simulink model "chart"  (R2020b)
settings: Solver=FixedStepDiscrete  StartTime=0.0  StopTime=10.0  FixedStep=0.1  RelTol=1e-3  EnableMultiTasking=on
settings Model: Creator=Admin  LastModifiedBy=Admin
settings SolverCC: AutoInsertRateTranBlk=on
settings DataIOCC: LimitDataPoints=on
settings OptimizationCC: LifeSpan=inf
settings DebuggingCC: AllowSymbolicDim=off  SFUnexpectedBacktrackingDiag=warning  SFNoUnconditionalDefaultTransitionDiag=warning  SFExecutionAtInitializationDiag=none  ArithmeticOperatorsInVariantConditions=warning
settings SFSimCC: SimUseLocalCustomCode=off  CustomCodeUndefinedFunction=UseInterfaceOnly
settings RTWCC: RTWUseLocalCustomCode=off
settings CodeAppCC: StateflowObjectComments=on
settings GRTTargetCC: TargetLangStandard=C89/C90 (ANSI)
settings ConfigComp: CovMetricSettings=dw  CovSaveCumulativeToWorkspaceVar=on  CovSaveSingleToWorkspaceVar=on  CovExternalEMLEnable=off  CovSFcnEnable=off

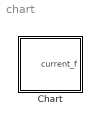
== system chart ==
  Chart : Stateflow chart  TreatAsAtomicUnit=on

== stateflow chart chart/Chart ==
  state LiftActive
    state Floor1
      entry:
      current_f=1;
    state Foor2
      entry:
      current_f=2;
    state Floor3
      entry:
      current_f=3;
    state Floor4
      entry:
      current_f=4;
    state Floor5
      entry:
      current_f=5;
    (default) -> Floor1
    Floor1 -> Foor2
    Foor2 -> Floor1 [order 2]
    Foor2 -> Floor3 [order 1]
    Floor3 -> Foor2 [order 1]
    Floor3 -> Floor4 [order 2]
    Floor4 -> Floor3 [order 1]
    Floor4 -> Floor5 [order 2]
    Floor5 -> Floor4
  state initial [group]
    state Idle
    state request
    (default) -> Idle
    Idle -> request : [request == 1]
  state Delay [group]
    state Dooropen
    state Doorclosed
    Doorclosed -> Dooropen
    Dooropen -> Doorclosed
  data: request local; current_f output
